simulink model "MotorDCControle"  (R2018a)
settings: Solver=VariableStepAuto  StartTime=0.0  StopTime=10  RelTol=1e-3
libraries: powerlib x6, powerlib_meascontrol x2, simulink x1
settings Model: Creator=MATHEUS  LastModifiedBy=MATHEUS

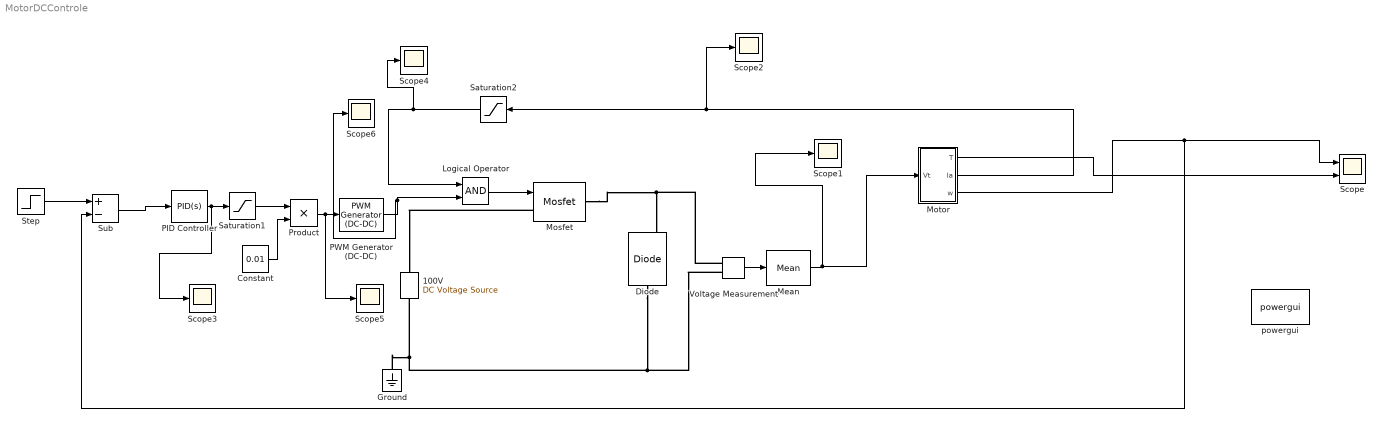
== system MotorDCControle ==
  100V : powerlib/Electrical Sources/DC Voltage Source  Amplitude=100  Measurements=None
  Constant : Constant  Value=0.01
  Diode : powerlib/Power Electronics/Diode  Ron=0.001  Lon=0  Vf=0.8  IC=0  UseSnubber=0  Rs=500  Cs=250e-9  Measurements=on
  Ground : powerlib/Elements/Ground  LConnTagsString=a
  Logical Operator : Logic  AllPortsSameDT=off  OutDataTypeStr=boolean
  Mean : powerlib_meascontrol/Measurements/Mean  Freq=60  Vinit=0  Ts=0
  Mosfet : powerlib/Power Electronics/Mosfet  Ron=0.1  Lon=0  Rd=0.01  Vfd=0  IC=0  Rs=1e5  Cs=inf  Measurements=off
  Motor : Subsystem
  PID Controller : simulink/Continuous/PID Controller  Controller=PID  TimeDomain=Continuous-time  SampleTime=-1  IntegratorMethod=Forward Euler  FilterMethod=Forward Euler  Form=Parallel  UseFilter=on  ControllerParametersSource=internal  P=0.05  I=3  D=1  N=100  InitialConditionSource=internal  InitialConditionForIntegrator=0  InitialConditionForFilter=0  ExternalReset=none  LimitOutput=off  UpperSaturationLimit=inf  LowerSaturationLimit=-inf  LinearizeAsGain=on  AntiWindupMode=none  Kb=1  TrackingMode=off  Kt=1  PParamMin=[]  PParamMax=[]  IParamMin=[]  IParamMax=[]  DParamMin=[]  DParamMax=[]  NParamMin=[]  NParamMax=[]  KbParamMin=[]  KbParamMax=[]  KtParamMin=[]  KtParamMax=[]  POutMin=[]  POutMax=[]  IOutMin=[]  IOutMax=[]  DOutMin=[]  DOutMax=[]  NOutMin=[]  NOutMax=[]  KbOutMin=[]  KbOutMax=[]  KtOutMin=[]  KtOutMax=[]  IntegratorOutMin=[]  IntegratorOutMax=[]  FilterOutMin=[]  FilterOutMax=[]  SumOutMin=[]  SumOutMax=[]  SumI1OutMin=[]  SumI1OutMax=[]  SumI2OutMin=[]  SumI2OutMax=[]  SumI3OutMin=[]  SumI3OutMax=[]  SumDOutMin=[]  SumDOutMax=[]  SaturationOutMin=[]  SaturationOutMax=[]  IntegratorContinuousStateAttributes=''  IntegratorStateMustResolveToSignalObject=off  IntegratorRTWStateStorageClass=Auto  FilterContinuousStateAttributes=''  FilterStateMustResolveToSignalObject=off  FilterRTWStateStorageClass=Auto  DifferentiatorICPrevScaledInput=0  DifferentiatorOutMin=[]  DifferentiatorOutMax=[]  FilterDiffOutCoefMin=[]  FilterDiffOutCoefMax=[]  SumDenOutMin=[]  SumDenOutMax=[]  SumNumOutMin=[]  SumNumOutMax=[]  ReciprocalOutMin=[]  ReciprocalOutMax=[]  DivideOutMin=[]  DivideOutMax=[]  TunerSelectOption=Transfer Function Based (PID Tuner App)
  PWM Generator (DC-DC) : powerlib_meascontrol/Pulse & Signal Generators/PWM Generator (DC-DC)  Fsw=5000  Ts=0
  Product : Product
  Saturation1 : Saturate  UpperLimit=1  LowerLimit=0
  Saturation2 : Saturate  UpperLimit=10  LowerLimit=0
  Scope : Scope  NumInputPorts=2
  Scope{1..6} (6 alike) : Scope
  Step : Step  Time=5  After=50  SampleTime=0
  "Sub " : Sum  Inputs=+-
  Voltage Measurement : powerlib/Measurements/Voltage Measurement  PhasorSimulation=off  OutputType=Complex  PSBequivalent=0
  powergui : powerlib/powergui  Priority=1  SimulationMode=Continuous  SampleTime=50e-6  frequency=60  Iterations=50  frequencyindice=0  Pbase=100e6  ErrMax=1e-4  UnitsV=kV  UnitsW=MW  buscounter=0  FunctionMessages=off  echomessages=off  EnableUseOfTLC=off  CurrentSourceSwitches=off  DisableSnubberDevices=off  DisableRonSwitches=off  DisableVfSwitches=off  DisplayEquations=off  SolverType=Tustin/Backward Euler (TBE)  Interpol=off  ExternalGateDelay=off  methode=off  Ts=100  x0status=blocks  SPID=off  SwTol=0  HookPort=off  RestoreLinks=warning  ResistiveCurrentMeasurement=off  Frange=[0:2:500]  Ylog=off  Xlog=on  ShowGrid=off  save=off  variable=ZData  structure=0  ZoomFFT=off  StartTime=0.0  cycles=1  DisplayStyle=1  fundamental=60  FreqAxis=off  MaxFrequency=1000  frequencyindicesteady=1  RmsSteady=1  display=off
  wires:
  "Sub "/1 -> PID Controller/1
  Step/1 -> "Sub "/1
  PID Controller/1 -> Scope3/1, Saturation1/1
  Voltage Measurement/1 -> Mean/1
  Mean/1 -> Motor/1(Vt), Scope1/1
  Motor/3(w) -> Scope/1, "Sub "/2
  Logical Operator/1 -> Mosfet/1
  PWM Generator (DC-DC)/1 -> Scope6/1, Logical Operator/2
  Motor/2(Ia) -> Scope2/1, Saturation2/1
  Saturation2/1 -> Scope4/1, Logical Operator/1
  Motor/1(T) -> Scope/2
  Saturation1/1 -> Product/1
  Product/1 -> Scope5/1, PWM Generator (DC-DC)/1
  Constant/1 -> Product/2
  connections:
  Voltage Measurement/LConn1 -- Mosfet/RConn1 -- Diode/RConn1
  Diode/LConn1 -- Ground/LConn1 -- 100V/LConn1 -- Voltage Measurement/LConn2
  Mosfet/LConn1 -- 100V/RConn1

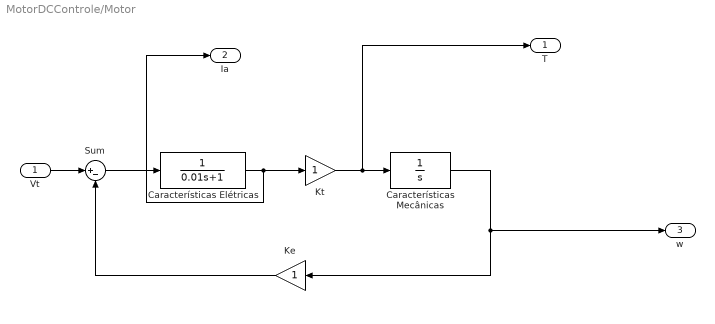
== system MotorDCControle/Motor ==
  Vt : Inport
  Características Elétricas : TransferFcn  Denominator=[0.01 1]
  "Características Mecânicas " : TransferFcn  Denominator=[1 0]
  Ke : Gain
  "Kt " : Gain
  Sum : Sum  Inputs=|+-
  T : Outport
  Ia : Outport  Port=2
  w : Outport  Port=3
  wires:
  "Características Mecânicas "/1 -> w/1, Ke/1
  "Kt "/1 -> T/1, "Características Mecânicas "/1
  Vt/1 -> Sum/1
  Ke/1 -> Sum/2
  Características Elétricas/1 -> Ia/1, "Kt "/1
  Sum/1 -> Características Elétricas/1
